simulink model "model"  (R2019b)
settings: Solver=VariableStepAuto  StartTime=0.0  StopTime=10.0  RelTol=1e-3
values from neighbouring files (symbols this model uses):
  cp = 1000    [WyznaczenieStatycznych.m]    (also in Wyznaczenie_K.m; onlyfp.m; state.m; transmitancja.m)
  Cvp = cp*ro_p*Vp    (= 240000)    [WyznaczenieStatycznych.m]    (also in Wyznaczenie_K.m; onlyfp.m; state.m; transmitancja.m)
  Cvw = cp*ro_p*Vw    (= 1200000)    [WyznaczenieStatycznych.m]    (also in Wyznaczenie_K.m = 360000; onlyfp.m = 360000; state.m = 360000; transmitancja.m = 360000)
  d_fp = 0    [WyznaczenieStatycznych.m]    (also in Wyznaczenie_K.m = 0.1; onlyfp.m = 0.5)
  d_Tz = 0    [WyznaczenieStatycznych.m]    (also in Wyznaczenie_K.m; onlyfp.m; state.m; transmitancja.m)
  d_Tzew = 0    [WyznaczenieStatycznych.m]    (also in Wyznaczenie_K.m; onlyfp.m; state.m = 3; transmitancja.m = 3)
  fp0 = fpN    (= 1)    [WyznaczenieStatycznych.m]    (also in Wyznaczenie_K.m = vfp0(i); onlyfp.m = vfp0(i))
  K1 = X(1)    [WyznaczenieStatycznych.m]    (also in Wyznaczenie_K.m; onlyfp.m; state.m; transmitancja.m)
  Kp = X(2)*a    [WyznaczenieStatycznych.m]    (also in Wyznaczenie_K.m; onlyfp.m; state.m; transmitancja.m)
  Kw = X(2)    [WyznaczenieStatycznych.m]    (also in Wyznaczenie_K.m; onlyfp.m; state.m; transmitancja.m)
  ro_p = 1.2    [WyznaczenieStatycznych.m]    (also in Wyznaczenie_K.m; onlyfp.m; state.m; transmitancja.m)
  t_skok = 100    [WyznaczenieStatycznych.m]    (also in Wyznaczenie_K.m = 500; onlyfp.m = 500; state.m = 500; transmitancja.m = 500)
  Tp0 = TpN    (= 18)    [WyznaczenieStatycznych.m]    (also in Wyznaczenie_K.m = Y(2); onlyfp.m = Y(2); state.m = Y(2); transmitancja.m = Y(2))
  Twew0 = TwewN    (= 22)    [WyznaczenieStatycznych.m]    (also in Wyznaczenie_K.m = Y(1); onlyfp.m = Y(1); state.m = Y(1); transmitancja.m = Y(1))
  Tz0 = TzN    (= 30)    [WyznaczenieStatycznych.m]    (also in Wyznaczenie_K.m = vTz0(i); onlyfp.m = vTz0(i); state.m = vTz0(i); transmitancja.m = vTz0(i))
  Tzew0 = TzewN    (= -2)    [WyznaczenieStatycznych.m]    (also in Wyznaczenie_K.m = vTzew0(i); onlyfp.m = vTzew0(i); state.m = vTzew0(i); transmitancja.m = vTzew0(i))
settings Model: Creator=Mariusz  LastModifiedBy=Mariusz

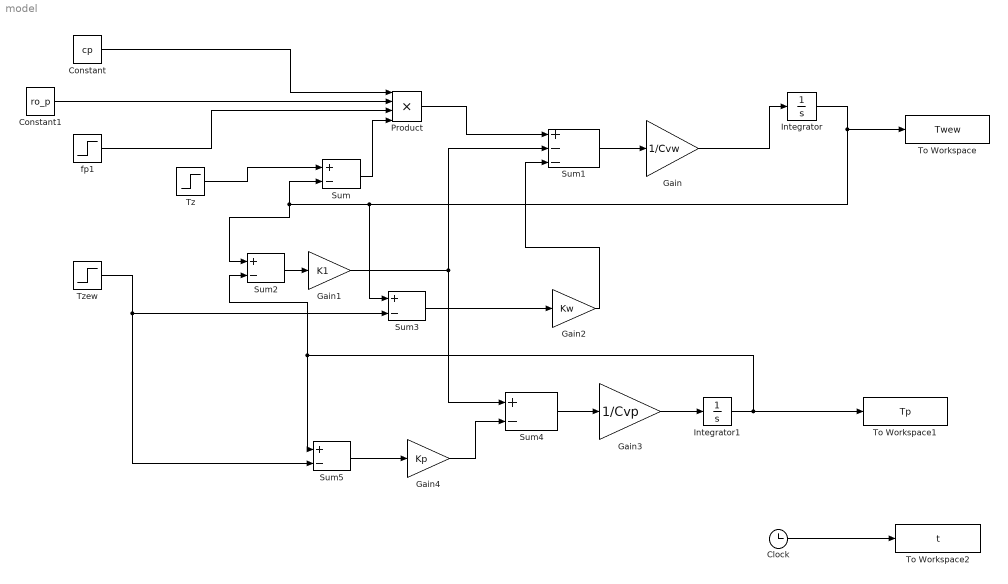
== system model ==
  Clock : Clock
  Constant : Constant  Value=cp
  Constant1 : Constant  Value=ro_p
  Gain : Gain  Gain=1/Cvw
  Gain1 : Gain  Gain=K1
  Gain2 : Gain  Gain=Kw
  Gain3 : Gain  Gain=1/Cvp
  Gain4 : Gain  Gain=Kp
  Integrator : Integrator  InitialCondition=Twew0
  Integrator1 : Integrator  InitialCondition=Tp0
  Product : Product  Inputs=4
  Sum{,2..5} (5 alike) : Sum  Inputs=+-
  Sum1 : Sum  Inputs=+--
  To Workspace : ToWorkspace  VariableName=Twew  SampleTime=-1
  To Workspace1 : ToWorkspace  VariableName=Tp  SampleTime=-1
  To Workspace2 : ToWorkspace  VariableName=t  SampleTime=-1
  Tz : Step  Time=t_skok  Before=Tz0  After=Tz0+ d_Tz  SampleTime=0
  Tzew : Step  Time=t_skok  Before=Tzew0  After=Tzew0 + d_Tzew  SampleTime=0  VectorParams1D=off  ZeroCross=off
  fp1 : Step  Time=t_skok  Before=fp0  After=fp0+d_fp  SampleTime=0
  wires:
  Gain/1 -> Integrator/1
  Constant/1 -> Product/1
  Constant1/1 -> Product/2
  fp1/1 -> Product/3
  Sum/1 -> Product/4
  Tz/1 -> Sum/1
  Integrator/1 -> To Workspace/1, Sum3/1, Sum/2, Sum2/1
  Sum1/1 -> Gain/1
  Product/1 -> Sum1/1
  Gain1/1 -> Sum1/2, Sum4/1
  Sum2/1 -> Gain1/1
  Integrator1/1 -> Sum5/1, Sum2/2, To Workspace1/1
  Gain2/1 -> Sum1/3
  Sum3/1 -> Gain2/1
  Tzew/1 -> Sum5/2, Sum3/2
  Gain3/1 -> Integrator1/1
  Gain4/1 -> Sum4/2
  Sum5/1 -> Gain4/1
  Sum4/1 -> Gain3/1
  Clock/1 -> To Workspace2/1
